simulink model "AdaptiveControl_DCAL"  (R2018a)
settings: Solver=ode45  StartTime=0.0  StopTime=60  RelTol=1e-3
values from neighbouring files (symbols this model uses):
  gam1 = 20    [AdaptiveControl2DOF.m]    (also in INV.m = asin( (a2*sin(Q2))/L ); INV_2DOF.m = asin( (a2*sin(Q2(k)))/L ); INV_2DOF_5thOrder.m = asin( (a2*sin(Q2(k)))/L ); INV_2DOF_Path.m = asin( (a2*sin(Q2(k)))/L ))
  gam2 = 20    [AdaptiveControl2DOF.m]    (also in INV_2DOF.m = acos( (a2^2 - L^2 - a1^2)/(-2*L*a1) ); INV_2DOF_Path.m = acos( (a2^2 - L^2 - a1^2)/(-2*L*a1) ))
  ka = 20    [AdaptiveControl2DOF.m]
  kp1 = 1.5    [AdaptiveControl2DOF.m]
  kp2 = 20.0    (= 20)    [AdaptiveControl2DOF.m]
  kv1 = 0.2    [AdaptiveControl2DOF.m]
  kv2 = 0.2    [AdaptiveControl2DOF.m]
  omega = 0.5    [AdaptiveControl2DOF.m]    (also in ComputedTorqueControl_2DOF.m = 1)
  the1 = theta1    (= 0.959931088597)    [AdaptiveControl2DOF.m]    (also in ComputedTorqueControl_2DOF.m = 0.523598775598)
  the2 = theta2    (= -0.959931088597)    [AdaptiveControl2DOF.m]    (also in ComputedTorqueControl_2DOF.m = 0.392699081699)
  tick = 0.002    [AdaptiveControl2DOF.m]    (also in ComputedTorqueControl_2DOF.m = 0.02)
libraries: dsppolyfun x2, simulink x2
settings Model: Creator=rashe  LastModifiedBy=rashe
settings SolverCC: ZeroCrossAlgorithm=Adaptive
settings DebuggingCC: MaxConsecutiveZCsMsg=none

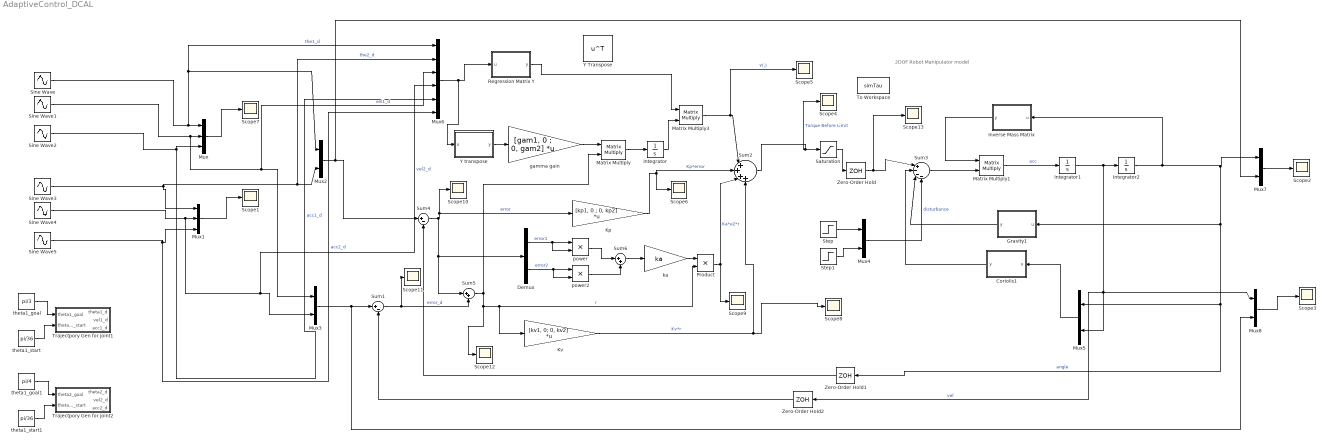
== system AdaptiveControl_DCAL ==
  note: 2DOF Robot Manipulator model
  Coriolis1 : MATLAB Function  TreatAsAtomicUnit=on
  Demux : Demux  Outputs=2
  Gravity1 : MATLAB Function  TreatAsAtomicUnit=on
  Integrator : Integrator  InitialCondition=[0; 0]
  Integrator1 : Integrator  InitialCondition=[0; 0]
  Integrator2 : Integrator  InitialCondition=[0; 0]
  Inverse Mass Matrix : MATLAB Function  TreatAsAtomicUnit=on
  Kp : Gain  Gain=[kp1, 0 ; 0, kp2]  Multiplication=Matrix(K*u)
  Kv : Gain  Gain=[kv1, 0; 0, kv2]  Multiplication=Matrix(K*u)
  Matrix Multiply : Product  Multiplication=Matrix(*)
  Matrix Multiply1 : Product  Multiplication=Matrix(*)
  Matrix Multiply3 : Product  Multiplication=Matrix(*)
  Mux : Mux  Inputs=3
  Mux1 : Mux  Inputs=3
  Mux{2..5,7..8} (6 alike) : Mux  Inputs=2
  Mux6 : Mux  Inputs=6
  Product : Product
  Regression Matrix Y : MATLAB Function  TreatAsAtomicUnit=on
  Saturation : Saturate  UpperLimit=4  LowerLimit=-4  LinearizeAsGain=off  ZeroCross=off
  Scope{1..13} (13 alike) : Scope
  Sine Wave : Sin  Amplitude=the1  Frequency=omega  Phase=pi/2  SampleTime=tick
  Sine Wave1 : Sin  Amplitude=-the1*omega  Frequency=omega  SampleTime=tick
  Sine Wave2 : Sin  Amplitude=-the1*omega^2  Frequency=omega  Phase=pi/2  SampleTime=tick
  Sine Wave3 : Sin  Amplitude=the2  Frequency=omega  Phase=pi/2  SampleTime=tick
  Sine Wave4 : Sin  Amplitude=-the2*omega  Frequency=omega  SampleTime=tick
  Sine Wave5 : Sin  Amplitude=-the2*omega^2  Frequency=omega  Phase=pi/2  SampleTime=tick
  Step : Step  Time=15  After=0.5  SampleTime=0
  Step1 : Step  Time=10  After=0.5  SampleTime=0
  Sum1 : Sum  Inputs=|+-
  Sum2 : Sum  Inputs=|++++
  Sum3 : Sum  Inputs=|+---
  Sum4 : Sum  Inputs=|+-
  Sum5 : Sum  Inputs=|++
  Sum6 : Sum  Inputs=|++
  To Workspace : ToWorkspace  VariableName=simTau  SaveFormat=Timeseries  SampleTime=tick
  Trajectpory Gen for joint1 : Subsystem
  Trajectpory Gen for joint2 : Subsystem
  Y Transpose : Math  Operator=transpose  SaturateOnIntegerOverflow=on
  Y transpose : MATLAB Function  TreatAsAtomicUnit=on
  Zero-Order Hold : ZeroOrderHold  SampleTime=tick
  Zero-Order Hold1 : ZeroOrderHold  SampleTime=tick
  Zero-Order Hold2 : ZeroOrderHold  SampleTime=tick
  gamma gain : Gain  Gain=[gam1, 0 ; 0, gam2]  Multiplication=Matrix(K*u)
  ka : Gain  Gain=ka
  power : Product
  "power2 " : Product
  theta1_goal : Constant  Value=pi/3  SampleTime=tick
  theta1_goal1 : Constant  Value=pi/4  SampleTime=tick
  theta1_start : Constant  Value=pi/36  SampleTime=tick
  theta1_start1 : Constant  Value=pi/36  SampleTime=tick
  wires:
  theta1_start1/1 -> Trajectpory Gen for joint2/2(theta2_start)
  theta1_start/1 -> Trajectpory Gen for joint1/2(theta1_start)
  Mux1/1 -> Scope1/1
  Mux/1 -> Scope7/1
  theta1_goal1/1 -> Trajectpory Gen for joint2/1(theta2_goal)
  theta1_goal/1 -> Trajectpory Gen for joint1/1(theta1_goal)
  Integrator2/1 -> Mux7/1, Zero-Order Hold1/1, Mux5/1, Gravity1/1(u), Inverse Mass Matrix/1(u)  "angle"
  Gravity1/1(y) -> Sum3/3
  Matrix Multiply1/1 -> Integrator1/1  "acc"
  Coriolis1/1(y) -> Sum3/2
  Inverse Mass Matrix/1(y) -> Matrix Multiply1/1
  Mux5/1 -> Coriolis1/1(u)
  Integrator1/1 -> Zero-Order Hold2/1, Mux8/1, Mux5/2, Integrator2/1  "vel"
  Sum3/1 -> Matrix Multiply1/2
  Mux6/1 -> Y transpose/1(u), Regression Matrix Y/1(u)
  Regression Matrix Y/1(y) -> Matrix Multiply3/1
  Mux2/1 -> Mux7/2, Sum4/1
  Mux3/1 -> Mux8/2, Sum1/1
  Sum4/1 -> Scope10/1, Kp/1, Sum5/1, Demux/1  "error"
  Kv/1 -> Scope8/1, Sum2/4  "Kv*r"
  Kp/1 -> Scope6/1, Sum2/2  "Kp*error"
  Sum1/1 -> Scope11/1, Sum5/2  "error_d"
  Sum5/1 -> Scope12/1, Product/2, Kv/1, Matrix Multiply/2  "r"
  gamma gain/1 -> Matrix Multiply/1
  Demux/1 -> power/2, power/1  "error1"
  Demux/2 -> "power2 "/2, "power2 "/1  "error2"
  power/1 -> Sum6/1
  "power2 "/1 -> Sum6/2
  Sum6/1 -> ka/1
  ka/1 -> Product/1
  Product/1 -> Sum2/3, Scope9/1  "Ka*e2*r"
  Matrix Multiply/1 -> Integrator/1
  Integrator/1 -> Matrix Multiply3/2
  Matrix Multiply3/1 -> Sum2/1, Scope5/1  "Y(.)"
  Mux7/1 -> Scope2/1
  Mux8/1 -> Scope3/1
  Step/1 -> Mux4/1
  Step1/1 -> Mux4/2
  Sine Wave/1 -> Mux6/1, Mux2/1, Mux/1  "the1_d"
  Sine Wave1/1 -> Mux6/3, Mux3/1, Mux/2  "vel1_d"
  Sine Wave2/1 -> Mux6/5, Mux/3  "acc1_d"
  Sine Wave5/1 -> Mux6/6, Mux1/3  "acc2_d"
  Sine Wave4/1 -> Mux6/4, Mux3/2, Mux1/2  "vel2_d"
  Sine Wave3/1 -> Mux1/1, Mux6/2, Mux2/2  "the2_d"
  Mux4/1 -> Sum3/4  "disturbance"
  Y transpose/1(y) -> gamma gain/1
  Sum2/1 -> Saturation/1, Scope4/1  "Torque Before Limit"
  Zero-Order Hold/1 -> Scope13/1, Sum3/1
  Saturation/1 -> Zero-Order Hold/1
  Zero-Order Hold1/1 -> Sum4/2
  Zero-Order Hold2/1 -> Sum1/2

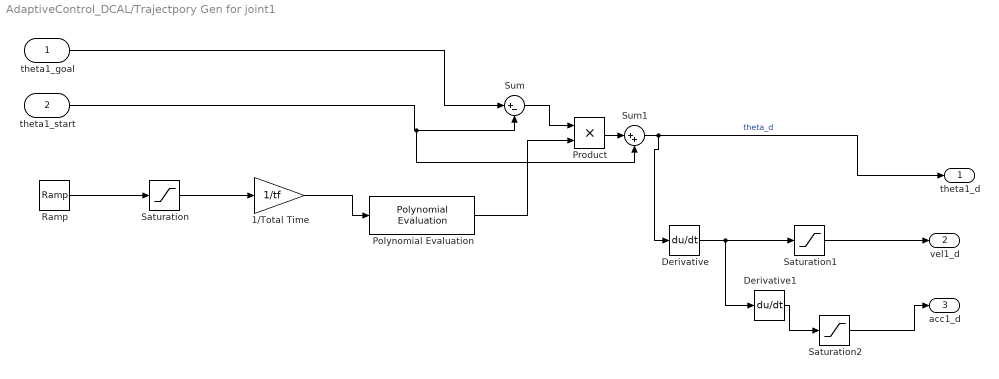
== system AdaptiveControl_DCAL/Trajectpory Gen for joint1 ==
  theta1_goal : Inport
  theta1_start : Inport  Port=2
  "1/Total Time " : Gain  Gain=1/tf
  Derivative : Derivative
  Derivative1 : Derivative
  Polynomial Evaluation : dsppolyfun/Polynomial Evaluation  useConstCoeffs=on  constCoeffs=[6 -15 10 0 0 0]
      settings: SourceProductName=DSP System Toolbox  SourceProductBaseCode=DS
  Product : Product
  Ramp : simulink/Sources/Ramp  slope=1  start=0  InitialOutput=0
  Saturation : Saturate  UpperLimit=tf  LowerLimit=-tf
  Saturation1 : Saturate  UpperLimit=5  LowerLimit=-5  ZeroCross=off
  Saturation2 : Saturate  UpperLimit=5  LowerLimit=-5  ZeroCross=off
  Sum : Sum  Inputs=|+-
  Sum1 : Sum  Inputs=|++
  theta1_d : Outport
  vel1_d : Outport  Port=2
  acc1_d : Outport  Port=3
  wires:
  Sum/1 -> Product/1
  Sum1/1 -> Derivative/1, theta1_d/1  "theta_d"
  Polynomial Evaluation/1 -> Product/2
  Ramp/1 -> Saturation/1
  "1/Total Time "/1 -> Polynomial Evaluation/1
  Saturation/1 -> "1/Total Time "/1
  Product/1 -> Sum1/1
  theta1_goal/1 -> Sum/1
  theta1_start/1 -> Sum1/2, Sum/2
  Derivative/1 -> Derivative1/1, Saturation1/1
  Derivative1/1 -> Saturation2/1
  Saturation1/1 -> vel1_d/1
  Saturation2/1 -> acc1_d/1

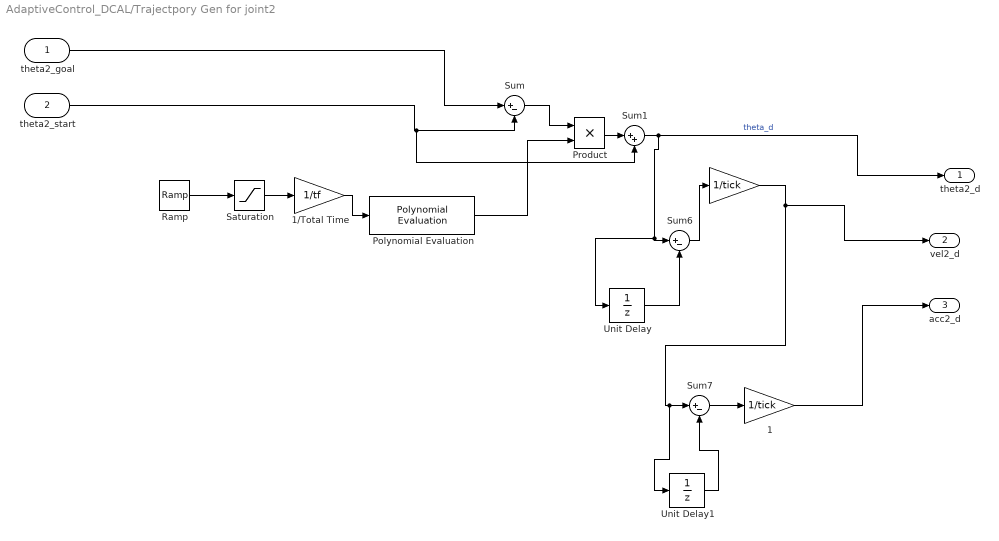
== system AdaptiveControl_DCAL/Trajectpory Gen for joint2 ==
  theta2_goal : Inport
  theta2_start : Inport  Port=2
  " " : Gain  Gain=1/tick
  " 1" : Gain  Gain=1/tick
  "1/Total Time " : Gain  Gain=1/tf
  Polynomial Evaluation : dsppolyfun/Polynomial Evaluation  useConstCoeffs=on  constCoeffs=[6 -15 10 0 0 0]
      settings: SourceProductName=DSP System Toolbox  SourceProductBaseCode=DS
  Product : Product
  Ramp : simulink/Sources/Ramp  slope=1  start=0  InitialOutput=0
  Saturation : Saturate  UpperLimit=tf  LowerLimit=-tf
  Sum : Sum  Inputs=|+-
  Sum1 : Sum  Inputs=|++
  Sum6 : Sum  Inputs=|+-
  Sum7 : Sum  Inputs=|+-
  Unit Delay : UnitDelay  SampleTime=tick
  Unit Delay1 : UnitDelay  SampleTime=tick
  theta2_d : Outport
  vel2_d : Outport  Port=2
  acc2_d : Outport  Port=3
  wires:
  Sum6/1 -> " "/1
  Sum/1 -> Product/1
  Sum1/1 -> theta2_d/1, Unit Delay/1, Sum6/1  "theta_d"
  " "/1 -> vel2_d/1, Unit Delay1/1, Sum7/1
  Polynomial Evaluation/1 -> Product/2
  Sum7/1 -> " 1"/1
  Unit Delay1/1 -> Sum7/2
  Ramp/1 -> Saturation/1
  "1/Total Time "/1 -> Polynomial Evaluation/1
  Saturation/1 -> "1/Total Time "/1
  Unit Delay/1 -> Sum6/2
  Product/1 -> Sum1/1
  " 1"/1 -> acc2_d/1
  theta2_goal/1 -> Sum/1
  theta2_start/1 -> Sum1/2, Sum/2

== matlab function AdaptiveControl_DCAL/Y transpose ==
  data: u input; y output
function y = fcn(u)

% Parameters
m1 = 0.233;   %kg
m2 = 0.2;
l1 = 0.192;
l2 = 0.185;
L1 = 0.27;
L2 = 0.23;
g = 9.81;

I1 = m1*l1^2;
I2 = m2*l2^2;

% Inputs
q1 = u(1);
q2 = u(2);

q1d = u(3);
q2d = u(4);

q1dd = u(5);
q2dd = u(6);

Y11 = l1^2*q1dd + l1^2*q1dd + g*l1*cos(q1);
Y12 = (L1^2 + l2^2 + L1*l2*cos(q2))*q1dd + l2^2*q1dd + (l2^2 + L1*l2*cos(q2))*q2dd + l2^2*q2dd - (L1*l2*sin(q2)*(q1d*q2d + 0.5*q2d^2)) + g*L1*cos(q1) + g*l2*cos(q1+q2);
Y21 = 0;
Y22 = (l2^2 + L1*l2*cos(q2))*q1dd + l2^2*q1dd + l2^2*q2dd + l2^2*q2dd + 0.5*L1*l2*sin(q2)*q1d^2 + g*l2*cos(q1+q2);


y = [Y11, Y21; Y12, Y22];

== matlab function AdaptiveControl_DCAL/Regression Matrix Y ==
  data: u input; y output
function y = Y(u)

% Parameters
m1 = 0.233;   %kg
m2 = 0.2;
l1 = 0.192;
l2 = 0.185;
L1 = 0.27;
L2 = 0.23;
g = 9.81;

I1 = m1*l1^2;
I2 = m2*l2^2;

% Inputs
q1 = u(1);
q2 = u(2);

q1d = u(3);
q2d = u(4);

q1dd = u(5);
q2dd = u(6);

Y11 = l1^2*q1dd + l1^2*q1dd + g*l1*cos(q1);
Y12 = (L1^2 + l2^2 + L1*l2*cos(q2))*q1dd + l2^2*q1dd + (l2^2 + L1*l2*cos(q2))*q2dd + l2^2*q2dd - (L1*l2*sin(q2)*(q1d*q2d + 0.5*q2d^2)) + g*L1*cos(q1) + g*l2*cos(q1+q2);
Y21 = 0;
Y22 = (l2^2 + L1*l2*cos(q2))*q1dd + l2^2*q1dd + l2^2*q2dd + l2^2*q2dd + 0.5*L1*l2*sin(q2)*q1d^2 + g*l2*cos(q1+q2);


y = [Y11, Y12; Y21, Y22];

== matlab function AdaptiveControl_DCAL/Inverse Mass Matrix ==
  data: u input; y output
function y = INVMass(u)

the1 = u(1);
the2 = u(2);

m1 = 0.233;   %kg     % True mass
m2 = 0.2;             % True mass
%m1 = 0.26;   %kg      % Unknown mass 
%m2 = 0.15;              % Unknown mass 
%l1 = 0.23;    % chagne the parameter value for make an imperfect model
%l2 = 0.17;    % chagne the parameter value for make an imperfect model
%L1 = 0.3;     % chagne the parameter value for make an imperfect model
l1 = 0.192;  % This is perferct parameter for perfect model
l2 = 0.185; % This is perferct parameter for perfect model
L1 = 0.27;   % This is perferct parameter for perfect model
L2 = 0.23;
g = 9.81;

I1 = m1*l1^2;
I2 = m2*l2^2;

M11 = m1*l1^2 + m2*(L1^2 + l2^2 + L1*l2*cos(the2)) + I1 + I2;
M12 = m2*(l2^2 + L1*l2*cos(the2)) + I2;
M21 = m2*(l2^2 + L1*l2*cos(the2)) + I2;
M22 = m2*l2^2 + I2;

coef = 1/(M11*M22 - M12*M21);
invM = coef*[M22, -M12; -M21, M11];

y = invM;

== matlab function AdaptiveControl_DCAL/Coriolis1 ==
  data: u input; y output
function y = V(u)

the1 = u(1);
the2 = u(2);

vel1 = u(3);
vel2 = u(4);

m1 = 0.233;   %kg     % True mass
m2 = 0.2;             % True mass
%m1 = 0.26;   %kg      % Unknown mass 
%m2 = 0.15;              % Unknown mass  
%l1 = 0.23;    % chagne the parameter value for make an imperfect model
%l2 = 0.17;    % chagne the parameter value for make an imperfect model
%L1 = 0.3;     % chagne the parameter value for make an imperfect model
l1 = 0.192;  % This is perferct parameter for perfect model
l2 = 0.185; % This is perferct parameter for perfect model
L1 = 0.27;   % This is perferct parameter for perfect model
L2 = 0.23;
g = 9.81;

I1 = m1*l1^2;
I2 = m2*l2^2;



V11 = -m2*L1*l2*sin(the2)*(vel1*vel2 + 0.5*vel2^2);
V21 = 0.5*m2*L1*l2*sin(the2)*vel1^2;


y = [V11;V21];

== matlab function AdaptiveControl_DCAL/Gravity1 ==
  data: u input; y output
function y = G(u)

the1 = u(1);
the2 = u(2);

m1 = 0.233;   %kg     % True mass
m2 = 0.2;             % True mass
%m1 = 0.26;   %kg      % Unknown mass 
%m2 = 0.15;              % Unknown mass 
%l1 = 0.23;    % chagne the parameter value for make an imperfect model
%l2 = 0.17;    % chagne the parameter value for make an imperfect model
%L1 = 0.3;     % chagne the parameter value for make an imperfect model
l1 = 0.192;  % This is perferct parameter for perfect model
l2 = 0.185; % This is perferct parameter for perfect model
L1 = 0.27;   % This is perferct parameter for perfect model
L2 = 0.23;
g = 9.81;

I1 = m1*l1^2;
I2 = m2*l2^2;

G11 = m1*g*l1*cos(the1) + m2*g*L1*cos(the1) + m2*g*l2*cos(the1+the2);
G21 = m2*g*l2*cos(the1+the2);

y = [G11;G21];
